simulink model "linear_control"  (R2023a)
settings: Solver=VariableStepAuto  StartTime=0.0  StopTime=10.0  RelTol=1e-3
settings Model: Creator=belov  LastModifiedBy=belov

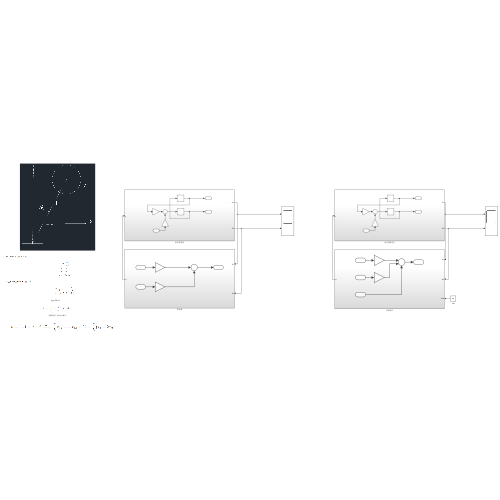
[thumbnail: Simulink's stored preview of the top-level diagram]
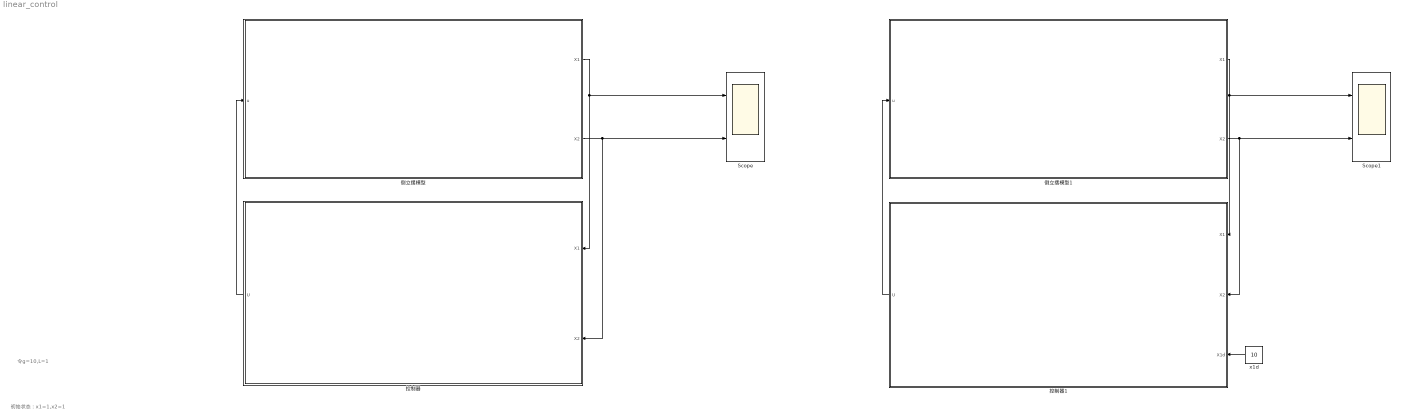
== system linear_control ==
  note: 初始状态：x1=1,x2=1
  note: 令g=10,L=1
  Scope : Scope  NumInputPorts=2
  Scope1 : Scope  NumInputPorts=2
  x1d : Constant  Value=10
  倒立摆模型 : Subsystem
  倒立摆模型1 : Subsystem
  控制器 : Subsystem
  控制器1 : Subsystem
  wires:
  倒立摆模型/1(X1) -> 控制器/1(X1), Scope/1
  倒立摆模型/2(X2) -> 控制器/2(X2), Scope/2
  控制器/1(U) -> 倒立摆模型/1(u)
  控制器1/1(U) -> 倒立摆模型1/1(u)
  倒立摆模型1/1(X1) -> 控制器1/1(X1), Scope1/1
  倒立摆模型1/2(X2) -> 控制器1/2(X2), Scope1/2
  x1d/1 -> 控制器1/3(X1d)

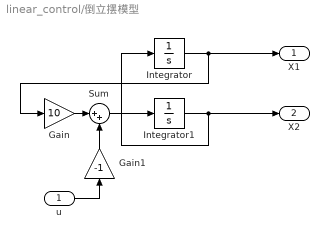
== system linear_control/倒立摆模型 ==
  u : Inport
  Gain : Gain  Gain=10
  Gain1 : Gain  Gain=-1
  Integrator : Integrator  InitialCondition=1
  Integrator1 : Integrator  InitialCondition=1
  Sum : Sum  Inputs=|++
  X1 : Outport
  X2 : Outport  Port=2
  wires:
  Gain1/1 -> Sum/2
  Integrator1/1 -> Integrator/1, X2/1
  Integrator/1 -> Gain/1, X1/1
  Sum/1 -> Integrator1/1
  Gain/1 -> Sum/1
  u/1 -> Gain1/1

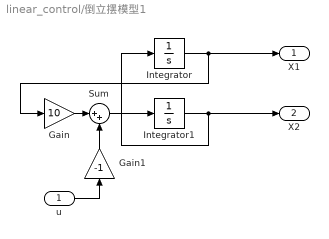
== system linear_control/倒立摆模型1 ==
  u : Inport
  Gain : Gain  Gain=10
  Gain1 : Gain  Gain=-1
  Integrator : Integrator
  Integrator1 : Integrator
  Sum : Sum  Inputs=|++
  X1 : Outport
  X2 : Outport  Port=2
  wires:
  u/1 -> Gain1/1
  Gain/1 -> Sum/1
  Sum/1 -> Integrator1/1
  Integrator/1 -> X1/1, Gain/1
  Integrator1/1 -> X2/1, Integrator/1
  Gain1/1 -> Sum/2

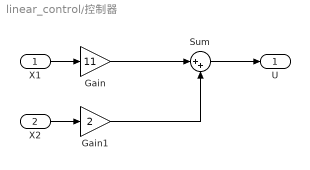
== system linear_control/控制器 ==
  X1 : Inport
  X2 : Inport  Port=2
  Gain : Gain  Gain=11
  Gain1 : Gain  Gain=2
  Sum : Sum  Inputs=|++
  U : Outport
  wires:
  X1/1 -> Gain/1
  X2/1 -> Gain1/1
  Sum/1 -> U/1
  Gain/1 -> Sum/1
  Gain1/1 -> Sum/2

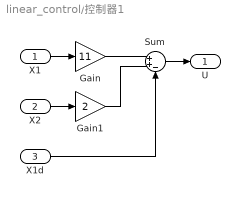
== system linear_control/控制器1 ==
  X1 : Inport
  X2 : Inport  Port=2
  X1d : Inport  Port=3
  Gain : Gain  Gain=11
  Gain1 : Gain  Gain=2
  Sum : Sum  Inputs=|++-
  U : Outport
  wires:
  X1d/1 -> Sum/3
  X1/1 -> Gain/1
  Gain/1 -> Sum/1
  X2/1 -> Gain1/1
  Gain1/1 -> Sum/2
  Sum/1 -> U/1
